simulink model "K_VALVE"  (Simulink 7.7)
settings: Solver=ode3  StartTime=0.0  StopTime=10.0  FixedStep=0.1  RelTol=1e-3
libraries: simulink x1
settings Model: Creator=danwheeler  LastModifiedBy=danwheeler
settings DataIOCC: ExternalInput=[t, u1, u2, u3, u4, u5, u6, u7, u8]  LoadExternalInput=on  SaveFinalState=on  SaveCompleteFinalSimState=on

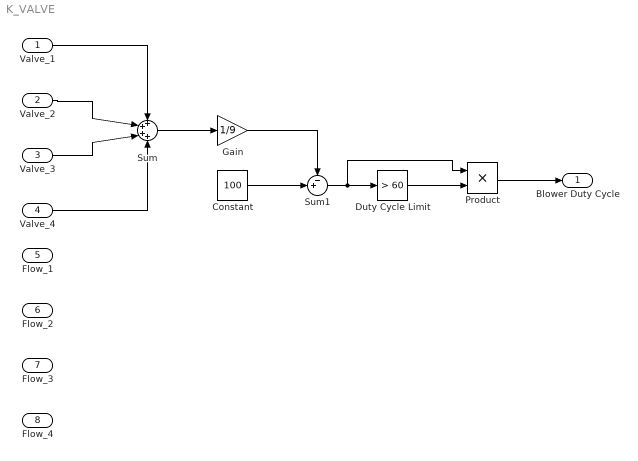
== system K_VALVE ==
  Valve_1 : Inport
  Valve_2 : Inport  Port=2
  Valve_3 : Inport  Port=3
  Valve_4 : Inport  Port=4
  Flow_1 : Inport  Port=5
  Flow_2 : Inport  Port=6
  Flow_3 : Inport  Port=7
  Flow_4 : Inport  Port=8
  Constant : Constant  Value=100
  Duty Cycle Limit : simulink/Logic and Bit Operations/Compare To Constant  SystemSampleTime=-1  relop=>  const=60  LogicOutDataTypeMode=uint8
  Gain : Gain  Gain=1/9
  Product : Product  RndMeth=Zero
  Sum : Sum  Inputs=++++
  Sum1 : Sum  Inputs=-+|
  Blower Duty Cycle : Outport
  wires:
  Valve_3/1 -> Sum/3
  Valve_2/1 -> Sum/2
  Valve_1/1 -> Sum/1
  Valve_4/1 -> Sum/4
  Sum/1 -> Gain/1
  Constant/1 -> Sum1/2
  Gain/1 -> Sum1/1
  Sum1/1 -> Duty Cycle Limit/1, Product/1
  Duty Cycle Limit/1 -> Product/2
  Product/1 -> Blower Duty Cycle/1
